simulink subsystem "HVDCPassThrough"  (R2024b)
settings: Solver=VariableStepAuto  StartTime=0.0  StopTime=10.0  RelTol=1e-3
settings Model: ModifiedByFormat=The MathWorks, Inc.  Creator=The MathWorks, Inc.  LastModifiedBy=The MathWorks, Inc.
settings SolverCC: MaxZcPerStep=1
settings DebuggingCC: UnconnectedInputMsg=warning  UnconnectedOutputMsg=warning  UnconnectedLineMsg=warning
settings ModelReferenceCC: EnableRefExpFcnMdlSchedulingChecks=on
settings RTWCC: GPUComputeCapability=3.5  DLArmComputeVersion=19.05

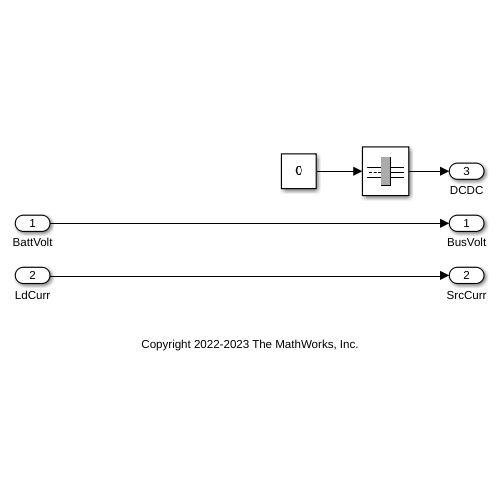
[thumbnail: Simulink's stored preview of the top-level diagram]
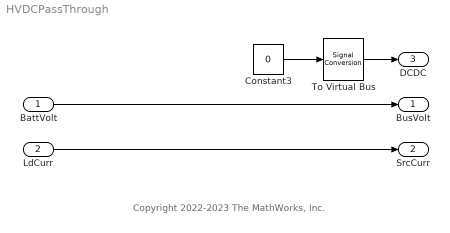
== system HVDCPassThrough ==
  note: Copyright 2022-2023 The MathWorks, Inc.
  BattVolt : Inport
  LdCurr : Inport  Port=2
  Constant3 : Constant  Value=0  OutDataTypeStr=Bus: DCDCBUS  SampleTime=Inf
  To Virtual Bus : SignalConversion  ConversionOutput=Virtual bus  OverrideOpt=off
  BusVolt : Outport  VectorParamsAs1DForOutWhenUnconnected=off
  SrcCurr : Outport  Port=2  VectorParamsAs1DForOutWhenUnconnected=off
  DCDC : Outport  Port=3
  wires:
  BattVolt/1 -> BusVolt/1
  LdCurr/1 -> SrcCurr/1
  To Virtual Bus/1 -> DCDC/1
  Constant3/1 -> To Virtual Bus/1
